simulink model "costasLoop"  (R2018b)
settings: Solver=FixedStepDiscrete  StartTime=0.0  StopTime=2000  RelTol=1e-3
libraries: simulink x2, commdigbbndpm3 x2, commfilt2 x2, dspstat3 x1, commrandsrc2 x1, commutil2 x1, commsink2 x1, commrflib2 x1
settings Model: Creator=sikor  LastModifiedBy=sikor
settings DataIOCC: LimitDataPoints=on  SaveFormat=Array
settings OptimizationCC: LifeSpan=inf
settings DebuggingCC: SolverPrmCheckMsg=warning  SFUnexpectedBacktrackingDiag=warning  SFNoUnconditionalDefaultTransitionDiag=warning
settings HardwareCC: ProdBitPerPointer=32  ProdBitPerSizeT=32  ProdBitPerPtrDiffT=32  ProdLargestAtomicFloat=None  ProdIntDivRoundTo=Undefined  ProdEndianess=Unspecified  ProdWordSize=32  ProdHWDeviceType=32-bit Generic
settings ModelReferenceCC: PropagateSignalLabelsOutOfModel=off
settings SFSimCC: SimUseLocalCustomCode=off
settings RTWCC: RTWUseLocalCustomCode=off
settings CodeAppCC: StateflowObjectComments=on
settings GRTTargetCC: TargetLangStandard=C89/C90 (ANSI)  GeneratePreprocessorConditionals=Disable all
settings ConfigComp: CovMetricSettings=dw  CovHtmlReporting=on  CovSaveCumulativeToWorkspaceVar=on  CovSaveSingleToWorkspaceVar=on  CovExternalEMLEnable=off  CovSFcnEnable=off

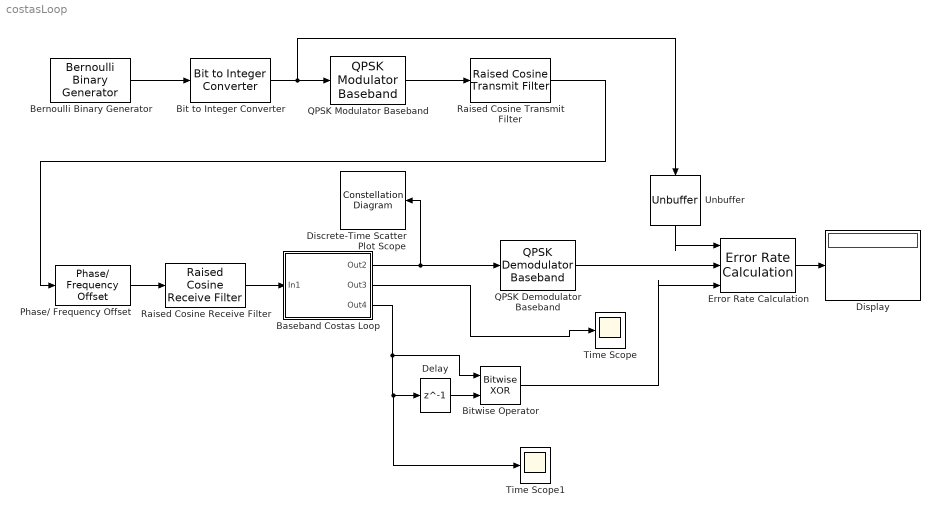
== system costasLoop ==
  Baseband Costas Loop : Subsystem  mask{loopBw=2.0*pi/100.0, sampleTime=1}
      mask prompts: loopBw "Select loop bandwidth"; sampleTime "Sample time"
      mask init:
      | damp=0.707;
      | %set_param('costasLoop','AlgebraicLoopSolver','TrustRegion')
      | alpha = (4.0 * damp * loopBw) / (1.0 + 2.0 * damp * loopBw + loopBw * loopBw); 
      | beta = (4.0 * loopBw * loopBw) / (1.0 + 2.0 * damp * loopBw + loopBw * loopBw); 
      | set_param(sprintf('%s/Baseband Costas Loop/Alfa',gcs),'Gain',sprintf('%f',alpha))
      | set_param(sprintf('%s/Baseband Costas Loop/Beta',gcs),'Gain',sprintf('%f',beta))
      | %set_param(sprintf('%s/Baseband Costas Loop/Mean1',gcs),'Ts',sprintf('%f',sampleTime))
      mask Display: disp('Costas\nLoop');
  Bernoulli Binary Generator : commrandsrc2/Bernoulli Binary Generator  P=0.5  seed=61  Ts=0.5  frameBased=on  sampPerFrame=2  orient=off  outDataType=boolean
      settings: SourceProductName=Communications Toolbox  SourceProductBaseCode=CM
  Bit to Integer Converter : commutil2/Bit to Integer Converter  nbits=2  bitOrder=MSB first  signedOutputValues=Unsigned  outDtype=int16  outDtypeSigned=Inherit via internal rule
      settings: SourceProductName=Communications Toolbox
  Bitwise Operator : simulink/Logic and Bit Operations/Bitwise Operator  logicop=XOR  UseBitMask=off  NumInputPorts=2  BitMask=bin2dec('11011001')  BitMaskRealWorld=Stored Integer
  Delay : Delay  DelayLength=1  InitialCondition=0
  Discrete-Time Scatter Plot Scope : ConstellationDiagram  Tag=ScatterPlot
  Display : Display
  Error Rate Calculation : commsink2/Error Rate Calculation  N=10  st_delay=0  cp_mode=Entire frame  subframe=[]  PMode=Port  WsName=ErrorVec  RsMode2=on  stop=off  numErr=100  maxBits=1e6
      settings: SourceProductName=Communications Toolbox
  Phase/ Frequency Offset : commrflib2/Phase// Frequency Offset  phaseOffset=20  freqPort=off  freqOffset=.000000045
      settings: SourceProductName=Communications Toolbox
  QPSK Demodulator Baseband : commdigbbndpm3/QPSK Demodulator Baseband  OutType=Integer  DecType=Hard decision  VarSource=Dialog  Variance=1  Dec=Gray  Ph=pi/4  outDtype1=Inherit via internal rule  outDtype2=int16  derotateFactorWordLen=16  derotateFactorDataTypeStr=Inherit: Same word length as input  derotateFactorLastDataTypeStr=Inherit: Same word length as input
      settings: SourceProductName=Communications Toolbox
  QPSK Modulator Baseband : commdigbbndpm3/QPSK Modulator Baseband  InType=Integer  Enc=Gray  Ph=pi/4  outDtype=double  outWordLen=16  outUDDataType=sfix(16)  outFracLenMode=Best precision  outFracLen=15  outDataTypeStr=double  outLastDataTypeStr=double
      settings: SourceProductName=Communications Toolbox
  Raised Cosine Receive Filter : commfilt2/Raised Cosine Receive Filter  filtType=Square root  R=0.2  filtSpan=10  N=4  downFactor=4  downOffset=0  filterGain=1  InputProcessing=Columns as channels (frame based)  RateOptions=Allow multirate processing  framing=Mute  checkCoeff=off  variableName=rcRxFilt  currentFiltSpan=10  D=5  inputOffset=0  sampMode=Mute  saveAsFlag=0  rateMode=Downsampling  checkGain=Normalized  launchFVT=on  roundingMode=Floor  overflowMode=off  coeffDataTypeStr=Inherit: Same word length as input  coeffMin=[]  coeffMax=[]  coeffLastDataTypeStr=Inherit: Same word length as input  accumDataTypeStr=Inherit: Same as product output  accumLastDataTypeStr=Inherit: Same as product output  outputDataTypeStr=Inherit: Same as accumulator  outputMin=[]  outputMax=[]  outputLastDataTypeStr=Inherit: Same as accumulator
      settings: SourceProductName=Communications Toolbox
  Raised Cosine Transmit Filter : commfilt2/Raised Cosine Transmit Filter  filtType=Square root  R=0.2  filtSpan=10  N=4  filterGain=1  InputProcessing=Columns as channels (frame based)  RateOptions=Allow multirate processing  framing=Mute  checkCoeff=off  variableName=rcTxFilt  checkGain=Normalized  sampMode=Mute  saveAsFlag=0  currentFiltSpan=10  D=5  launchFVT=on  roundingMode=Floor  overflowMode=off  coeffDataTypeStr=Inherit: Same word length as input  coeffMin=[]  coeffMax=[]  coeffLastDataTypeStr=Inherit: Same word length as input  outputDataTypeStr=Inherit: Same as accumulator  outputMin=[]  outputMax=[]  outputLastDataTypeStr=Inherit: Same as accumulator
      settings: SourceProductName=Communications Toolbox
  Time Scope : Scope
  Time Scope1 : Scope
  Unbuffer : Unbuffer
  wires:
  Bernoulli Binary Generator/1 -> Bit to Integer Converter/1
  Raised Cosine Transmit Filter/1 -> Phase/ Frequency Offset/1
  QPSK Modulator Baseband/1 -> Raised Cosine Transmit Filter/1
  Bit to Integer Converter/1 -> Unbuffer/1, QPSK Modulator Baseband/1
  Error Rate Calculation/1 -> Display/1
  QPSK Demodulator Baseband/1 -> Error Rate Calculation/2
  Phase/ Frequency Offset/1 -> Raised Cosine Receive Filter/1
  Raised Cosine Receive Filter/1 -> Baseband Costas Loop/1(In1)
  Baseband Costas Loop/1(Out2) -> Discrete-Time Scatter Plot Scope/1, QPSK Demodulator Baseband/1
  Baseband Costas Loop/2(Out3) -> Time Scope/1
  Delay/1 -> Bitwise Operator/2
  Baseband Costas Loop/3(Out4) -> Time Scope1/1, Delay/1, Bitwise Operator/1
  Bitwise Operator/1 -> Error Rate Calculation/3
  Unbuffer/1 -> Error Rate Calculation/1

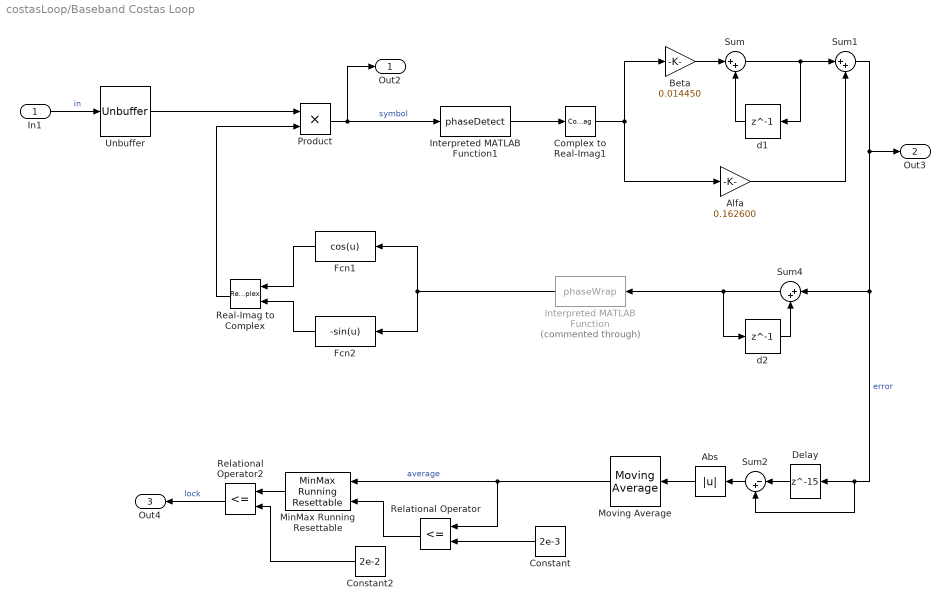
== system costasLoop/Baseband Costas Loop ==
  In1 : Inport
  Abs : Abs
  Alfa : Gain  Gain=0.162600
  Beta : Gain  Gain=0.014450
  Complex to Real-Imag1 : ComplexToRealImag  Output=Real
  Constant : Constant  Value=2e-3
  Constant2 : Constant  Value=2e-2
  Delay : Delay  DelayLength=15  InitialCondition=0
  Fcn1 : Fcn  Expr=cos(u)
  Fcn2 : Fcn  Expr=-sin(u)
  Interpreted MATLAB Function : MATLABFcn  Commented=through  MATLABFcn=phaseWrap
  Interpreted MATLAB Function1 : MATLABFcn  MATLABFcn=phaseDetect
  MinMax Running Resettable : simulink/Math Operations/MinMax Running Resettable  Function=max  vinit=0.0
  Moving Average : dspstat3/Moving Average  Method=Sliding window  ForgettingFactorPort=off  SpecifyWindowLength=on  WindowLength=32  ForgettingFactor=0.9  SimulateUsing=Code generation
  Product : Product  OutDataTypeStr=double  RndMeth=Round
  Real-Imag to Complex : RealImagToComplex
  Relational Operator : RelationalOperator  Operator=<=  OutDataTypeStr=boolean  RndMeth=Nearest
  Relational Operator2 : RelationalOperator  Operator=<=  OutDataTypeStr=boolean  RndMeth=Nearest
  Sum : Sum  Inputs=|++  OutDataTypeStr=double  RndMeth=Round
  Sum1 : Sum  Inputs=|++  OutDataTypeStr=double  RndMeth=Nearest
  Sum2 : Sum  Inputs=|-+
  Sum4 : Sum  Inputs=|++
  Unbuffer : Unbuffer
  d1 : Delay  DelayLength=1  InitialCondition=0
  d2 : Delay  DelayLength=1  InitialCondition=0
  Out2 : Outport
  Out3 : Outport  Port=2
  Out4 : Outport  Port=3
  wires:
  In1/1 -> Unbuffer/1  "in"
  d1/1 -> Sum/2
  Sum/1 -> d1/1, Sum1/1
  Alfa/1 -> Sum1/2
  Beta/1 -> Sum/1
  Product/1 -> Out2/1, Interpreted MATLAB Function1/1  "symbol"
  Real-Imag to Complex/1 -> Product/2
  Unbuffer/1 -> Product/1
  Sum4/1 -> d2/1, Interpreted MATLAB Function/1
  d2/1 -> Sum4/2
  Interpreted MATLAB Function/1 -> Fcn1/1, Fcn2/1
  Fcn1/1 -> Real-Imag to Complex/1
  Fcn2/1 -> Real-Imag to Complex/2
  Sum1/1 -> Sum2/2, Delay/1, Sum4/1, Out3/1  "error"
  Interpreted MATLAB Function1/1 -> Complex to Real-Imag1/1
  Complex to Real-Imag1/1 -> Alfa/1, Beta/1
  Constant2/1 -> Relational Operator2/2
  Delay/1 -> Sum2/1
  Constant/1 -> Relational Operator/2
  Sum2/1 -> Abs/1
  Moving Average/1 -> MinMax Running Resettable/1, Relational Operator/1  "average"
  Relational Operator/1 -> MinMax Running Resettable/2
  MinMax Running Resettable/1 -> Relational Operator2/1
  Abs/1 -> Moving Average/1
  Relational Operator2/1 -> Out4/1  "lock"
